simulink model "ass2model"  (R2015b)
settings: Solver=VariableStepDiscrete  StartTime=0.0  StopTime=24.0  MaxStep=0.48  RelTol=1e-3
undefined symbols (not defined in the file): sigbuilder_block
settings Model: Creator=straigchri  LastModifiedBy=straigchri

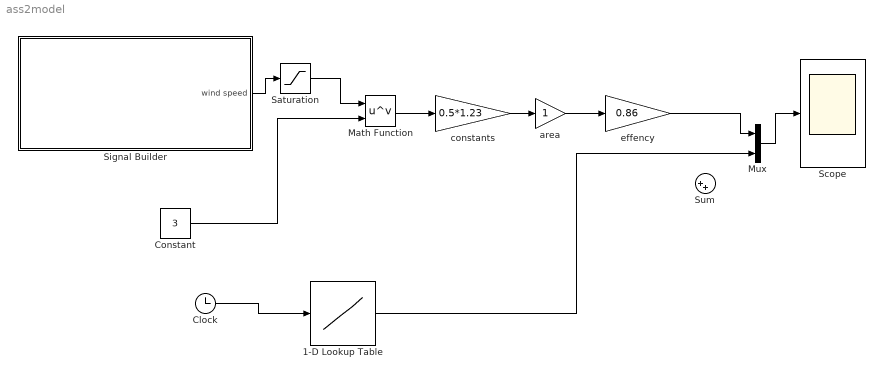
== system ass2model ==
  1-D Lookup Table : Lookup_n-D  NumberOfTableDimensions=1  BreakpointsForDimension1=[0,1,2,3,4,5]  Table=[2,2,4,9,9,6]  InternalRulePriority=Speed  RndMeth=Simplest  InputSameDT=on
  Clock : Clock
      settings: Decimation=24
  Constant : Constant  Value=3
  Math Function : Math  Operator=pow  SaturateOnIntegerOverflow=on
  Mux : Mux  Inputs=2
  Saturation : Saturate  UpperLimit=40  LowerLimit=0
  Scope : Scope
  Signal Builder : Subsystem  Tag=STV Subsys  LoadFcn=sigbuilder_block('load');  StartFcn=sigbuilder_block('start');  StopFcn=sigbuilder_block('stop');  ClipboardFcn=sigbuilder_block('clipboard');  mask(Sigbuilder block){}
      mask help: Simulink:masks:SigbuilderBlock_MD
      mask init:
      | if ~strcmp(get_param(bdroot(gcbh),'SimulationStatus'),'stopped') tuvar = sigbuilder_block('maskInit'); end
      settings: CopyFcn=sigbuilder_block('copy');  DeleteFcn=sigbuilder_block('delete');  ModelCloseFcn=sigbuilder_block('modelClose');  PreSaveFcn=sigbuilder_block('preSave');  PauseFcn=sigbuilder_block('pause');  ContinueFcn=sigbuilder_block('continue');  NameChangeFcn=sigbuilder_block('namechange');  OpenFcn=sigbuilder_block('open',[1.5 29.25 726 328.5 ]);  CloseFcn=sigbuilder_block('close');
      mask Display: plot(0, 0, 100, 100,[2, 2, 32, 32, 2], [68, 8, 8, 68, 68],[32, 2], [38, 38], [32, 19, 2],[53, 60, 44], [32, 17, 17, 2],[16, 16, 31, 31]);txt = getActiveGroup(gcbh);text(2, 100, txt,'verticalAlignment', 'top');
  Sum : Sum  Inputs=|++
  area : Gain
  constants : Gain  Gain=0.5*1.23
  effency : Gain  Gain=0.86
  wires:
  effency/1 -> Mux/1
  area/1 -> effency/1
  constants/1 -> area/1
  Math Function/1 -> constants/1
  Signal Builder/1(wind speed) -> Saturation/1
  Constant/1 -> Math Function/2
  Clock/1 -> 1-D Lookup Table/1
  1-D Lookup Table/1 -> Mux/2
  Mux/1 -> Scope/1
  Saturation/1 -> Math Function/1

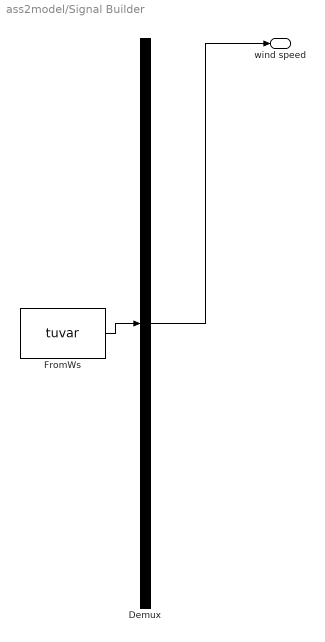
== system ass2model/Signal Builder ==
  Demux : Demux  Tag=STV Demux  Outputs=1
  FromWs : FromWorkspace  Tag=STV FromWs  VariableName=tuvar  SampleTime=0
      SigBuilderData=|
      | common.afterFinalStr = 'Extrapolate'
      | common.sampleTime = 0
      | dataSet.timeRange = [0 24]
      | dataSet.name = 'Group 1'
      | sbobj.Groups.Name = 'Group 1'
      | sbobj.Groups.Signals.Name = 'wind speed'
      | sbobj.Groups.Signals.XData = [0 0.9 1.5 2.35 2.65 3.3 3.95 6.2 7.75 10.95 12.5 14.1 14.7 16.55 19.3 21.25 24]
      | sbobj.Groups.Signals.YData = [14.65 19 24.6 27 30 35.2 41.2 36.4 41.8 37 32.4 26.8 20 15 22.4 12 15.4]
      | sbobj.Groups.TimeRange = [0 24]
  wind speed : Outport  Tag=STV Outport
  wires:
  Demux/1 -> wind speed/1
  FromWs/1 -> Demux/1
